simulink model "CompensatorModel"  (R2023b)
settings: Solver=VariableStepAuto  StartTime=0.0  StopTime=0.05  RelTol=1e-3
settings Model: Creator=sammasten  LastModifiedBy=sammasten

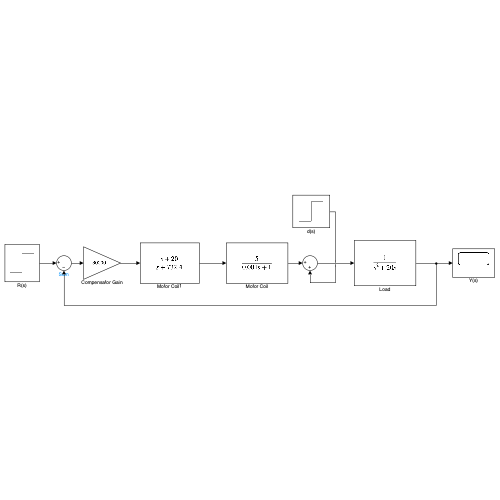
[thumbnail: Simulink's stored preview of the top-level diagram]
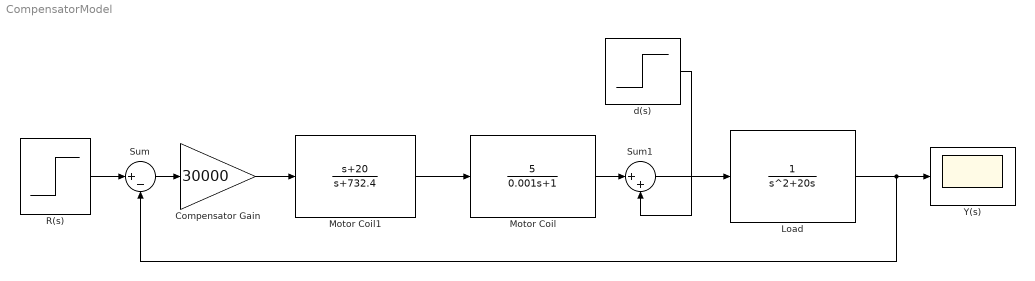
== system CompensatorModel ==
  Compensator Gain : Gain  Gain=30000
  Load : TransferFcn  Denominator=[1 20 0]
  Motor Coil : TransferFcn  Numerator=[5]  Denominator=[0.001 1]
  Motor Coil1 : TransferFcn  Numerator=[1 20]  Denominator=[1 732.4]
  R(s) : Step  Time=0.001  SampleTime=0
  Sum : Sum  Inputs=|+-
  Sum1 : Sum  Inputs=|++
  Y(s) : Scope
  d(s) : Step  SampleTime=0
  wires:
  Compensator Gain/1 -> Motor Coil1/1
  Motor Coil1/1 -> Motor Coil/1
  Motor Coil/1 -> Sum1/1
  Sum/1 -> Compensator Gain/1
  d(s)/1 -> Sum1/2
  Load/1 -> Sum/2, Y(s)/1
  R(s)/1 -> Sum/1
  Sum1/1 -> Load/1
